simulink model "tasukete"  (R2019b)
settings: Solver=VariableStepAuto  StartTime=0.0  StopTime=60  RelTol=1e-3
values from neighbouring files (symbols this model uses):
  a0 = 1.3    [mf.mat]    (also in model_2r.m; model_Fy.m)
  a1 = -0.0274    [mf.mat]    (also in model_2r.m; model_Fy.m)
  a10 = 0.015    [mf.mat]    (also in model_2r.m; model_Fy.m)
  a11 = 0.00849    [mf.mat]    (also in model_2r.m = 0.0849; model_Fy.m)
  a12 = -0.0103    [mf.mat]    (also in model_2r.m; model_Fy.m)
  a13 = 0.0395    [mf.mat]    (also in model_2r.m; model_Fy.m)
  a2 = 1.05    [mf.mat]    (also in model_2r.m; model_Fy.m)
  a3 = 1.18    [mf.mat]    (also in model_2r.m; model_Fy.m)
  a4 = 7.69    [mf.mat]    (also in model_2r.m; model_Fy.m)
  a5 = 0.009    [mf.mat]    (also in model_2r.m; model_Fy.m)
  a6 = -0.257    [mf.mat]    (also in model_2r.m; model_Fy.m)
  a7 = 0.224    [mf.mat]    (also in model_2r.m; model_Fy.m)
  a8 = 0.025    [mf.mat]    (also in model_2r.m; model_Fy.m)
  a9 = 0.01    [mf.mat]    (also in model_2r.m; model_Fy.m)
  g = 9.81    [mf.mat]    (also in model_2r.m)
  Iz = 1500    [mf.mat]    (also in model_2r.m)
  lf = 1.4    [mf.mat]    (also in model_2r.m = 1.2)
  lr = 1.2    [mf.mat]    (also in model_2r.m = 1.4)
  m = 1200    [mf.mat]    (also in model_2r.m)
  v = 8.33333333333    [mf.mat]    (also in model_2r.m = 100)
libraries: simulink_extras x1, simulink x1
settings Model: Creator=yknc1  LastModifiedBy=Peanatsu
settings SFSimCC: CustomCodeUndefinedFunction=UseInterfaceOnly

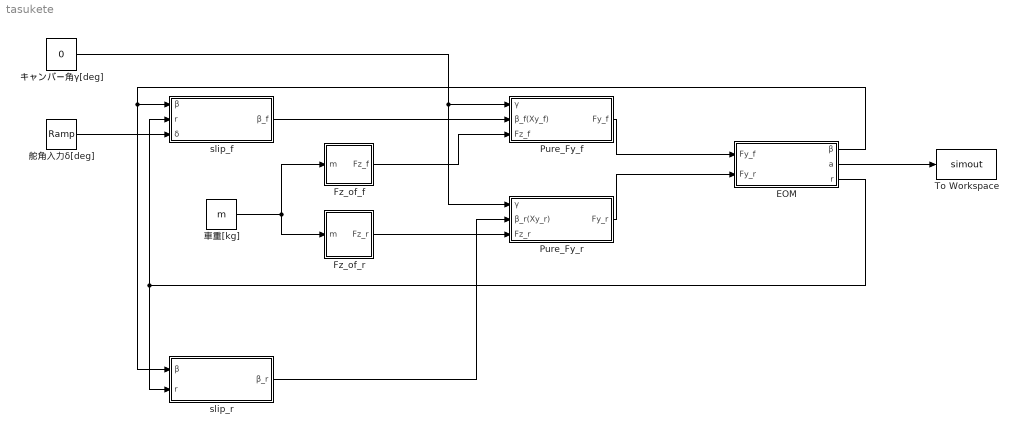
== system tasukete ==
  EOM : Subsystem
  Fz_of_f : Subsystem
  Fz_of_r : Subsystem
  Pure_Fy_f : Subsystem
  Pure_Fy_r : Subsystem
  To Workspace : ToWorkspace  VariableName=simout  SaveFormat=Timeseries  SampleTime=-1
  slip_f : Subsystem
  slip_r : Subsystem
  キャンバー角γ[deg] : Constant  Value=0
  舵角入力δ[deg] : simulink/Sources/Ramp  slope=5  start=0  InitialOutput=1
  車重[kg] : Constant  Value=m
  wires:
  キャンバー角γ[deg]/1 -> Pure_Fy_r/1(γ), Pure_Fy_f/1(γ)
  slip_f/1(β_f) -> Pure_Fy_f/2(β_f(Xy_f))
  slip_r/1(β_r) -> Pure_Fy_r/2(β_r(Xy_r))
  EOM/1(β) -> slip_f/1(β), slip_r/1(β)
  EOM/3(r) -> slip_r/2(r), slip_f/2(r)
  車重[kg]/1 -> Fz_of_r/1(m), Fz_of_f/1(m)
  Fz_of_f/1(Fz_f) -> Pure_Fy_f/3(Fz_f)
  Fz_of_r/1(Fz_r) -> Pure_Fy_r/3(Fz_r)
  Pure_Fy_r/1(Fy_r) -> EOM/2(Fy_r)
  Pure_Fy_f/1(Fy_f) -> EOM/1(Fy_f)
  EOM/2(a) -> To Workspace/1
  舵角入力δ[deg]/1 -> slip_f/3(δ)

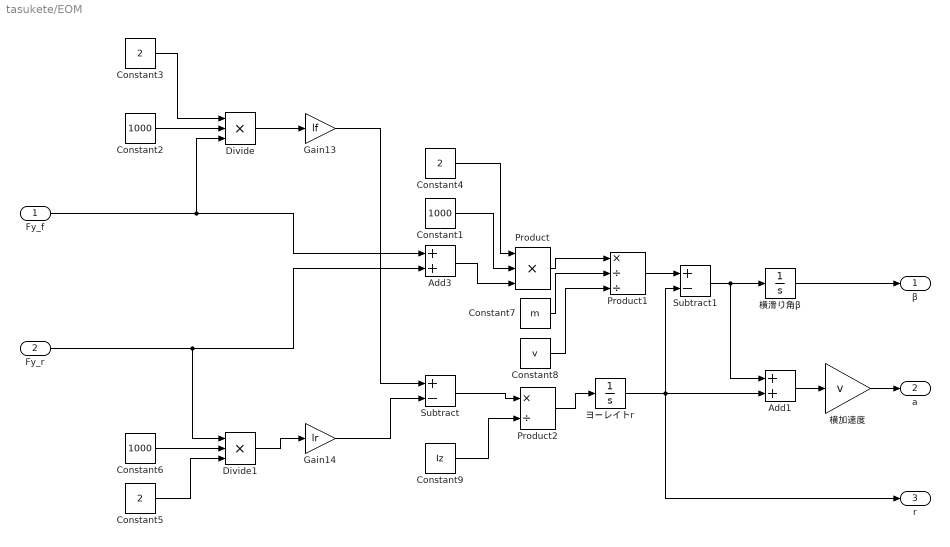
== system tasukete/EOM ==
  Fy_f : Inport
  Fy_r : Inport  Port=2
  Add1 : Sum
  Add3 : Sum
  Constant1 : Constant  Value=1000
  Constant2 : Constant  Value=1000
  Constant3 : Constant  Value=2
  Constant4 : Constant  Value=2
  Constant5 : Constant  Value=2
  Constant6 : Constant  Value=1000
  Constant7 : Constant  Value=m
  Constant8 : Constant  Value=v
  Constant9 : Constant  Value=Iz
  Divide : Product  Inputs=***
  Divide1 : Product  Inputs=***
  Gain13 : Gain  Gain=lf
  Gain14 : Gain  Gain=lr
  Product : Product  Inputs=3
  Product1 : Product  Inputs=*//
  Product2 : Product  Inputs=*/
  Subtract : Sum  Inputs=+-
  Subtract1 : Sum  Inputs=+-
  ヨーレイトr : Integrator
  横加速度 : Gain  Gain=v
  横滑り角β : Integrator
  β : Outport  VectorParamsAs1DForOutWhenUnconnected=off
  a : Outport  Port=2  VectorParamsAs1DForOutWhenUnconnected=off
  r : Outport  Port=3  VectorParamsAs1DForOutWhenUnconnected=off
  wires:
  Subtract1/1 -> Add1/1, 横滑り角β/1
  Constant5/1 -> Divide1/3
  Constant6/1 -> Divide1/2
  ヨーレイトr/1 -> Subtract1/2, Add1/2, r/1
  Divide/1 -> Gain13/1
  Constant1/1 -> Product/2
  Fy_r/1 -> Divide1/1, Add3/2
  Constant4/1 -> Product/1
  Constant2/1 -> Divide/2
  横滑り角β/1 -> β/1
  Add1/1 -> 横加速度/1
  Constant3/1 -> Divide/1
  横加速度/1 -> a/1
  Divide1/1 -> Gain14/1
  Add3/1 -> Product/3
  Gain14/1 -> Subtract/2
  Product1/1 -> Subtract1/1
  Gain13/1 -> Subtract/1
  Fy_f/1 -> Divide/3, Add3/1
  Subtract/1 -> Product2/1
  Product/1 -> Product1/1
  Constant8/1 -> Product1/3
  Constant7/1 -> Product1/2
  Product2/1 -> ヨーレイトr/1
  Constant9/1 -> Product2/2

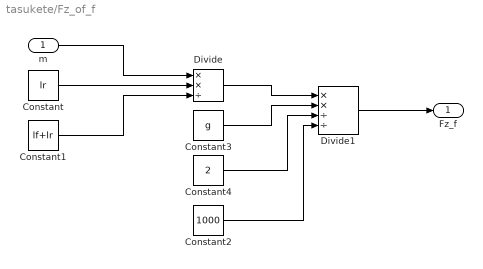
== system tasukete/Fz_of_f ==
  m : Inport
  Constant : Constant  Value=lr
  Constant1 : Constant  Value=lf+lr
  Constant2 : Constant  Value=1000
  Constant3 : Constant  Value=g
  Constant4 : Constant  Value=2
  Divide : Product  Inputs=**/
  Divide1 : Product  Inputs=**//
  Fz_f : Outport  VectorParamsAs1DForOutWhenUnconnected=off
  wires:
  m/1 -> Divide/1
  Constant/1 -> Divide/2
  Constant1/1 -> Divide/3
  Divide/1 -> Divide1/1
  Constant3/1 -> Divide1/2
  Constant4/1 -> Divide1/3
  Constant2/1 -> Divide1/4
  Divide1/1 -> Fz_f/1

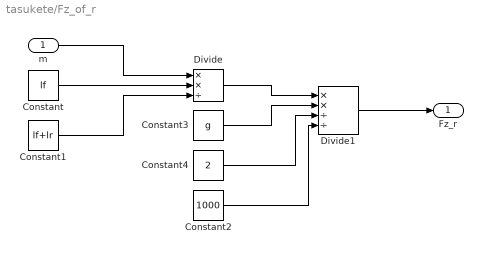
== system tasukete/Fz_of_r ==
  m : Inport
  Constant : Constant  Value=lf
  Constant1 : Constant  Value=lf+lr
  Constant2 : Constant  Value=1000
  Constant3 : Constant  Value=g
  Constant4 : Constant  Value=2
  Divide : Product  Inputs=**/
  Divide1 : Product  Inputs=**//
  Fz_r : Outport  VectorParamsAs1DForOutWhenUnconnected=off
  wires:
  Constant3/1 -> Divide1/2
  Divide1/1 -> Fz_r/1
  Constant/1 -> Divide/2
  Constant2/1 -> Divide1/4
  m/1 -> Divide/1
  Constant4/1 -> Divide1/3
  Constant1/1 -> Divide/3
  Divide/1 -> Divide1/1

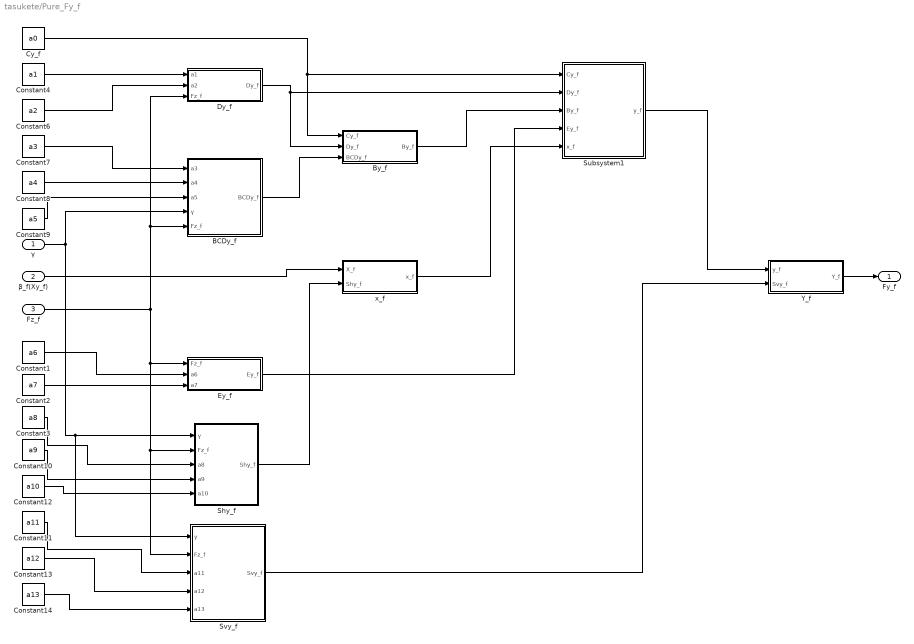
== system tasukete/Pure_Fy_f ==
  γ : Inport
  β_f(Xy_f) : Inport  Port=2
  Fz_f : Inport  Port=3
  BCDy_f : Subsystem
  By_f : Subsystem
  Constant1 : Constant  Value=a6
  Constant10 : Constant  Value=a9
  Constant11 : Constant  Value=a11
  Constant12 : Constant  Value=a10
  Constant13 : Constant  Value=a12
  Constant14 : Constant  Value=a13
  Constant2 : Constant  Value=a7
  Constant3 : Constant  Value=a8
  Constant4 : Constant  Value=a1
  Constant6 : Constant  Value=a2
  Constant7 : Constant  Value=a3
  Constant8 : Constant  Value=a4
  Constant9 : Constant  Value=a5
  Cy_f : Constant  Value=a0
  Dy_f : Subsystem
  Ey_f : Subsystem
  Shy_f : Subsystem
  Subsystem1 : Subsystem
  Svy_f : Subsystem
  Y_f : Subsystem
  x_f : Subsystem
  Fy_f : Outport  VectorParamsAs1DForOutWhenUnconnected=off
  wires:
  Constant4/1 -> Dy_f/1(a1)
  Constant6/1 -> Dy_f/2(a2)
  Fz_f/1 -> BCDy_f/5(Fz_f), Dy_f/3(Fz_f), Ey_f/1(Fz_f), Svy_f/2(Fz_f), Shy_f/2(Fz_f)
  Constant1/1 -> Ey_f/2(a6)
  Constant2/1 -> Ey_f/3(a7)
  γ/1 -> Shy_f/1(γ), Svy_f/1(γ), BCDy_f/4(γ)
  Constant3/1 -> Shy_f/3(a8)
  Constant10/1 -> Shy_f/4(a9)
  Constant12/1 -> Shy_f/5(a10)
  Constant11/1 -> Svy_f/3(a11)
  Constant13/1 -> Svy_f/4(a12)
  Constant14/1 -> Svy_f/5(a13)
  Constant7/1 -> BCDy_f/1(a3)
  Constant8/1 -> BCDy_f/2(a4)
  Constant9/1 -> BCDy_f/3(a5)
  Cy_f/1 -> By_f/1(Cy_f), Subsystem1/1(Cy_f)
  Dy_f/1(Dy_f) -> By_f/2(Dy_f), Subsystem1/2(Dy_f)
  BCDy_f/1(BCDy_f) -> By_f/3(BCDy_f)
  β_f(Xy_f)/1 -> x_f/1(X_f)
  Shy_f/1(Shy_f) -> x_f/2(Shy_f)
  By_f/1(By_f) -> Subsystem1/3(By_f)
  Ey_f/1(Ey_f) -> Subsystem1/4(Ey_f)
  x_f/1(x_f) -> Subsystem1/5(x_f)
  Subsystem1/1(y_f) -> Y_f/1(y_f)
  Svy_f/1(Svy_f) -> Y_f/2(Svy_f)
  Y_f/1(Y_f) -> Fy_f/1

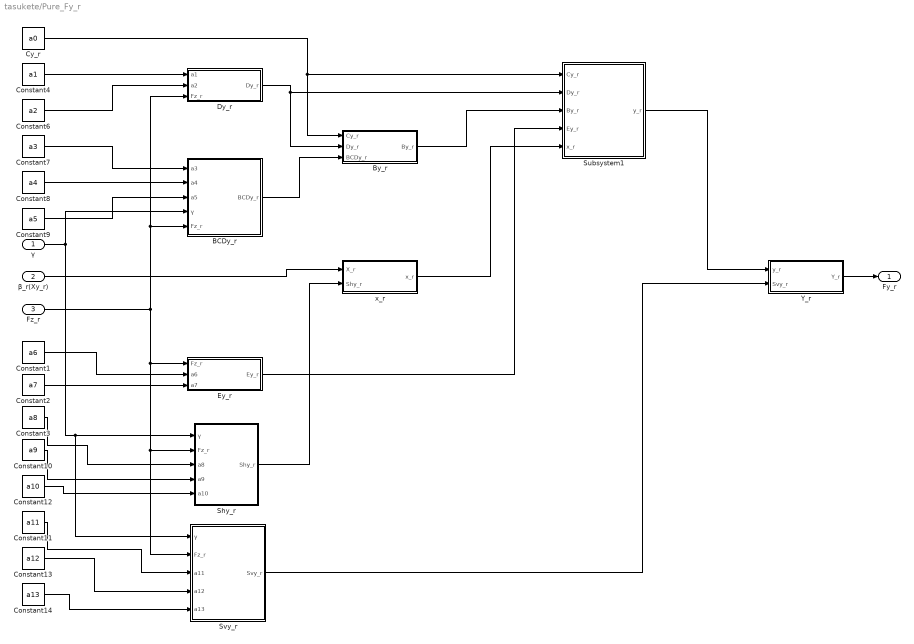
== system tasukete/Pure_Fy_r ==
  γ : Inport
  β_r(Xy_r) : Inport  Port=2
  Fz_r : Inport  Port=3
  BCDy_r : Subsystem
  By_r : Subsystem
  Constant1 : Constant  Value=a6
  Constant10 : Constant  Value=a9
  Constant11 : Constant  Value=a11
  Constant12 : Constant  Value=a10
  Constant13 : Constant  Value=a12
  Constant14 : Constant  Value=a13
  Constant2 : Constant  Value=a7
  Constant3 : Constant  Value=a8
  Constant4 : Constant  Value=a1
  Constant6 : Constant  Value=a2
  Constant7 : Constant  Value=a3
  Constant8 : Constant  Value=a4
  Constant9 : Constant  Value=a5
  Cy_r : Constant  Value=a0
  Dy_r : Subsystem
  Ey_r : Subsystem
  Shy_r : Subsystem
  Subsystem1 : Subsystem
  Svy_r : Subsystem
  Y_r : Subsystem
  x_r : Subsystem
  Fy_r : Outport  VectorParamsAs1DForOutWhenUnconnected=off
  wires:
  Constant4/1 -> Dy_r/1(a1)
  Constant6/1 -> Dy_r/2(a2)
  Fz_r/1 -> BCDy_r/5(Fz_r), Dy_r/3(Fz_r), Ey_r/1(Fz_r), Svy_r/2(Fz_r), Shy_r/2(Fz_r)
  Constant1/1 -> Ey_r/2(a6)
  Constant2/1 -> Ey_r/3(a7)
  γ/1 -> Shy_r/1(γ), Svy_r/1(γ), BCDy_r/4(γ)
  Constant3/1 -> Shy_r/3(a8)
  Constant10/1 -> Shy_r/4(a9)
  Constant12/1 -> Shy_r/5(a10)
  Constant11/1 -> Svy_r/3(a11)
  Constant13/1 -> Svy_r/4(a12)
  Constant14/1 -> Svy_r/5(a13)
  Constant7/1 -> BCDy_r/1(a3)
  Constant8/1 -> BCDy_r/2(a4)
  Constant9/1 -> BCDy_r/3(a5)
  Cy_r/1 -> By_r/1(Cy_r), Subsystem1/1(Cy_r)
  Dy_r/1(Dy_r) -> By_r/2(Dy_r), Subsystem1/2(Dy_r)
  BCDy_r/1(BCDy_r) -> By_r/3(BCDy_r)
  β_r(Xy_r)/1 -> x_r/1(X_r)
  Shy_r/1(Shy_r) -> x_r/2(Shy_r)
  By_r/1(By_r) -> Subsystem1/3(By_r)
  Ey_r/1(Ey_r) -> Subsystem1/4(Ey_r)
  x_r/1(x_r) -> Subsystem1/5(x_r)
  Subsystem1/1(y_r) -> Y_r/1(y_r)
  Svy_r/1(Svy_r) -> Y_r/2(Svy_r)
  Y_r/1(Y_r) -> Fy_r/1

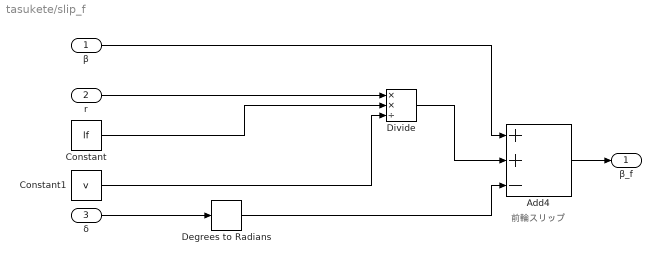
== system tasukete/slip_f ==
  note: 前輪スリップ
  β : Inport
  r : Inport  Port=2
  δ : Inport  Port=3
  Add4 : Sum  Inputs=++-
  Constant : Constant  Value=lf
  Constant1 : Constant  Value=v
  Degrees to Radians : simulink_extras/Transformations/Degrees to Radians
  Divide : Product  Inputs=**/
  β_f : Outport  VectorParamsAs1DForOutWhenUnconnected=off
  wires:
  Add4/1 -> β_f/1
  β/1 -> Add4/1
  δ/1 -> Degrees to Radians/1
  Degrees to Radians/1 -> Add4/3
  r/1 -> Divide/1
  Constant/1 -> Divide/2
  Constant1/1 -> Divide/3
  Divide/1 -> Add4/2

== system tasukete/slip_r ==
  β : Inport
  r : Inport  Port=2
  Constant : Constant  Value=lr
  Constant1 : Constant  Value=v
  Divide : Product  Inputs=**/
  Subtract : Sum  Inputs=+-
  β_r : Outport  VectorParamsAs1DForOutWhenUnconnected=off
  wires:
  β/1 -> Subtract/1
  r/1 -> Divide/1
  Subtract/1 -> β_r/1
  Constant/1 -> Divide/2
  Constant1/1 -> Divide/3
  Divide/1 -> Subtract/2

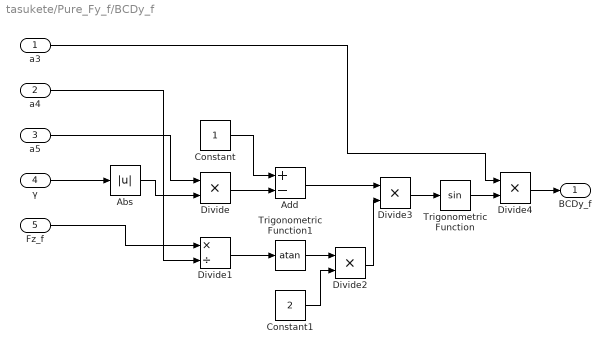
== system tasukete/Pure_Fy_f/BCDy_f ==
  a3 : Inport
  a4 : Inport  Port=2
  a5 : Inport  Port=3
  γ : Inport  Port=4
  Fz_f : Inport  Port=5
  Abs : Abs
  Add : Sum  Inputs=+-
  Constant : Constant
  Constant1 : Constant  Value=2
  Divide{,2..4} (4 alike) : Product  Inputs=**
  Divide1 : Product  Inputs=*/
  Trigonometric Function : Trigonometry
  Trigonometric Function1 : Trigonometry  Operator=atan
  BCDy_f : Outport  VectorParamsAs1DForOutWhenUnconnected=off
  wires:
  γ/1 -> Abs/1
  Abs/1 -> Divide/2
  a5/1 -> Divide/1
  Constant/1 -> Add/1
  Divide/1 -> Add/2
  Fz_f/1 -> Divide1/1
  a4/1 -> Divide1/2
  Divide1/1 -> Trigonometric Function1/1
  Trigonometric Function1/1 -> Divide2/1
  Constant1/1 -> Divide2/2
  Add/1 -> Divide3/1
  Divide2/1 -> Divide3/2
  Divide3/1 -> Trigonometric Function/1
  a3/1 -> Divide4/1
  Trigonometric Function/1 -> Divide4/2
  Divide4/1 -> BCDy_f/1

== system tasukete/Pure_Fy_f/By_f ==
  Cy_f : Inport
  Dy_f : Inport  Port=2
  BCDy_f : Inport  Port=3
  Divide : Product  Inputs=*//
  By_f : Outport  VectorParamsAs1DForOutWhenUnconnected=off
  wires:
  BCDy_f/1 -> Divide/1
  Dy_f/1 -> Divide/2
  Cy_f/1 -> Divide/3
  Divide/1 -> By_f/1

== system tasukete/Pure_Fy_f/Dy_f ==
  a1 : Inport
  a2 : Inport  Port=2
  Fz_f : Inport  Port=3
  Product : Product
  Product1 : Product
  μy_f : Sum
  Dy_f : Outport  VectorParamsAs1DForOutWhenUnconnected=off
  wires:
  a1/1 -> Product/1
  Fz_f/1 -> Product1/2, Product/2
  a2/1 -> μy_f/1
  Product/1 -> μy_f/2
  μy_f/1 -> Product1/1
  Product1/1 -> Dy_f/1

== system tasukete/Pure_Fy_f/Ey_f ==
  Fz_f : Inport
  a6 : Inport  Port=2
  a7 : Inport  Port=3
  Add : Sum
  Product : Product
  Ey_f : Outport  VectorParamsAs1DForOutWhenUnconnected=off
  wires:
  Fz_f/1 -> Product/1
  a6/1 -> Product/2
  Product/1 -> Add/1
  a7/1 -> Add/2
  Add/1 -> Ey_f/1

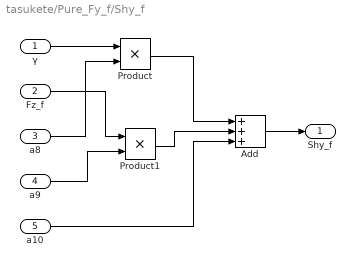
== system tasukete/Pure_Fy_f/Shy_f ==
  γ : Inport
  Fz_f : Inport  Port=2
  a8 : Inport  Port=3
  a9 : Inport  Port=4
  a10 : Inport  Port=5
  Add : Sum  Inputs=+++
  Product : Product
  Product1 : Product
  Shy_f : Outport  VectorParamsAs1DForOutWhenUnconnected=off
  wires:
  γ/1 -> Product/1
  a8/1 -> Product/2
  a9/1 -> Product1/2
  Fz_f/1 -> Product1/1
  a10/1 -> Add/3
  Product1/1 -> Add/2
  Product/1 -> Add/1
  Add/1 -> Shy_f/1

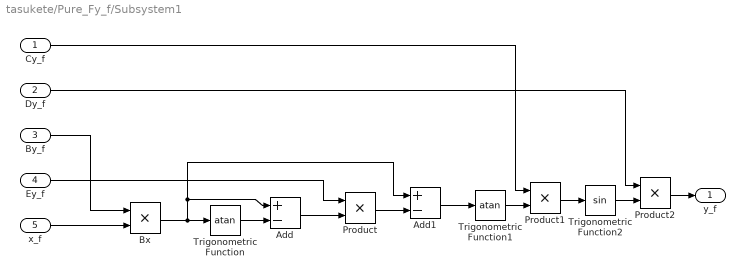
== system tasukete/Pure_Fy_f/Subsystem1 ==
  Cy_f : Inport
  Dy_f : Inport  Port=2
  By_f : Inport  Port=3
  Ey_f : Inport  Port=4
  x_f : Inport  Port=5
  Add : Sum  Inputs=+-
  Add1 : Sum  Inputs=+-
  Bx : Product
  Product : Product
  Product1 : Product
  Product2 : Product
  Trigonometric Function : Trigonometry  Operator=atan
  Trigonometric Function1 : Trigonometry  Operator=atan
  Trigonometric Function2 : Trigonometry
  y_f : Outport  VectorParamsAs1DForOutWhenUnconnected=off
  wires:
  x_f/1 -> Bx/2
  By_f/1 -> Bx/1
  Bx/1 -> Add1/1, Add/1, Trigonometric Function/1
  Trigonometric Function/1 -> Add/2
  Add/1 -> Product/2
  Ey_f/1 -> Product/1
  Product/1 -> Add1/2
  Add1/1 -> Trigonometric Function1/1
  Trigonometric Function1/1 -> Product1/2
  Cy_f/1 -> Product1/1
  Product1/1 -> Trigonometric Function2/1
  Trigonometric Function2/1 -> Product2/2
  Dy_f/1 -> Product2/1
  Product2/1 -> y_f/1

== system tasukete/Pure_Fy_f/Svy_f ==
  γ : Inport
  Fz_f : Inport  Port=2
  a11 : Inport  Port=3
  a12 : Inport  Port=4
  a13 : Inport  Port=5
  Add : Sum  Inputs=+++
  Product : Product  Inputs=3
  Product1 : Product
  Svy_f : Outport  VectorParamsAs1DForOutWhenUnconnected=off
  wires:
  γ/1 -> Product/1
  Fz_f/1 -> Product1/1, Product/2
  a11/1 -> Product/3
  a12/1 -> Product1/2
  Product/1 -> Add/1
  Product1/1 -> Add/2
  a13/1 -> Add/3
  Add/1 -> Svy_f/1

== system tasukete/Pure_Fy_f/Y_f ==
  y_f : Inport
  Svy_f : Inport  Port=2
  Add : Sum
  Y_f : Outport  VectorParamsAs1DForOutWhenUnconnected=off
  wires:
  Add/1 -> Y_f/1
  Svy_f/1 -> Add/2
  y_f/1 -> Add/1

== system tasukete/Pure_Fy_f/x_f ==
  X_f : Inport
  Shy_f : Inport  Port=2
  Add : Sum
  x_f : Outport  VectorParamsAs1DForOutWhenUnconnected=off
  wires:
  X_f/1 -> Add/1
  Shy_f/1 -> Add/2
  Add/1 -> x_f/1

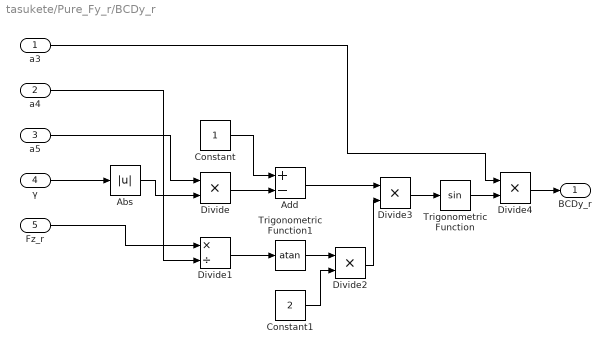
== system tasukete/Pure_Fy_r/BCDy_r ==
  a3 : Inport
  a4 : Inport  Port=2
  a5 : Inport  Port=3
  γ : Inport  Port=4
  Fz_r : Inport  Port=5
  Abs : Abs
  Add : Sum  Inputs=+-
  Constant : Constant
  Constant1 : Constant  Value=2
  Divide{,2..4} (4 alike) : Product  Inputs=**
  Divide1 : Product  Inputs=*/
  Trigonometric Function : Trigonometry
  Trigonometric Function1 : Trigonometry  Operator=atan
  BCDy_r : Outport  VectorParamsAs1DForOutWhenUnconnected=off
  wires:
  γ/1 -> Abs/1
  Abs/1 -> Divide/2
  a5/1 -> Divide/1
  Constant/1 -> Add/1
  Divide/1 -> Add/2
  Fz_r/1 -> Divide1/1
  a4/1 -> Divide1/2
  Divide1/1 -> Trigonometric Function1/1
  Trigonometric Function1/1 -> Divide2/1
  Constant1/1 -> Divide2/2
  Add/1 -> Divide3/1
  Divide2/1 -> Divide3/2
  Divide3/1 -> Trigonometric Function/1
  a3/1 -> Divide4/1
  Trigonometric Function/1 -> Divide4/2
  Divide4/1 -> BCDy_r/1

== system tasukete/Pure_Fy_r/By_r ==
  Cy_r : Inport
  Dy_r : Inport  Port=2
  BCDy_r : Inport  Port=3
  Divide : Product  Inputs=*//
  By_r : Outport  VectorParamsAs1DForOutWhenUnconnected=off
  wires:
  BCDy_r/1 -> Divide/1
  Dy_r/1 -> Divide/2
  Cy_r/1 -> Divide/3
  Divide/1 -> By_r/1

== system tasukete/Pure_Fy_r/Dy_r ==
  a1 : Inport
  a2 : Inport  Port=2
  Fz_r : Inport  Port=3
  Product : Product
  Product1 : Product
  μy_r : Sum
  Dy_r : Outport  VectorParamsAs1DForOutWhenUnconnected=off
  wires:
  a1/1 -> Product/1
  Fz_r/1 -> Product1/2, Product/2
  a2/1 -> μy_r/1
  Product/1 -> μy_r/2
  μy_r/1 -> Product1/1
  Product1/1 -> Dy_r/1

== system tasukete/Pure_Fy_r/Ey_r ==
  Fz_r : Inport
  a6 : Inport  Port=2
  a7 : Inport  Port=3
  Add : Sum
  Product : Product
  Ey_r : Outport  VectorParamsAs1DForOutWhenUnconnected=off
  wires:
  Fz_r/1 -> Product/1
  a6/1 -> Product/2
  Product/1 -> Add/1
  a7/1 -> Add/2
  Add/1 -> Ey_r/1

== system tasukete/Pure_Fy_r/Shy_r ==
  γ : Inport
  Fz_r : Inport  Port=2
  a8 : Inport  Port=3
  a9 : Inport  Port=4
  a10 : Inport  Port=5
  Add : Sum  Inputs=+++
  Product : Product
  Product1 : Product
  Shy_r : Outport  VectorParamsAs1DForOutWhenUnconnected=off
  wires:
  γ/1 -> Product/1
  a8/1 -> Product/2
  a9/1 -> Product1/2
  Fz_r/1 -> Product1/1
  a10/1 -> Add/3
  Product1/1 -> Add/2
  Product/1 -> Add/1
  Add/1 -> Shy_r/1

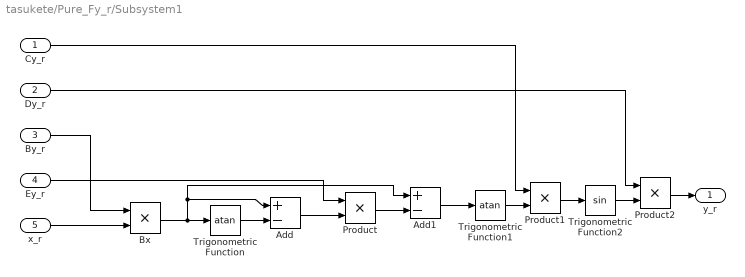
== system tasukete/Pure_Fy_r/Subsystem1 ==
  Cy_r : Inport
  Dy_r : Inport  Port=2
  By_r : Inport  Port=3
  Ey_r : Inport  Port=4
  x_r : Inport  Port=5
  Add : Sum  Inputs=+-
  Add1 : Sum  Inputs=+-
  Bx : Product
  Product : Product
  Product1 : Product
  Product2 : Product
  Trigonometric Function : Trigonometry  Operator=atan
  Trigonometric Function1 : Trigonometry  Operator=atan
  Trigonometric Function2 : Trigonometry
  y_r : Outport  VectorParamsAs1DForOutWhenUnconnected=off
  wires:
  x_r/1 -> Bx/2
  By_r/1 -> Bx/1
  Bx/1 -> Add1/1, Add/1, Trigonometric Function/1
  Trigonometric Function/1 -> Add/2
  Add/1 -> Product/2
  Ey_r/1 -> Product/1
  Product/1 -> Add1/2
  Add1/1 -> Trigonometric Function1/1
  Trigonometric Function1/1 -> Product1/2
  Cy_r/1 -> Product1/1
  Product1/1 -> Trigonometric Function2/1
  Trigonometric Function2/1 -> Product2/2
  Dy_r/1 -> Product2/1
  Product2/1 -> y_r/1

== system tasukete/Pure_Fy_r/Svy_r ==
  γ : Inport
  Fz_r : Inport  Port=2
  a11 : Inport  Port=3
  a12 : Inport  Port=4
  a13 : Inport  Port=5
  Add : Sum  Inputs=+++
  Product : Product  Inputs=3
  Product1 : Product
  Svy_r : Outport  VectorParamsAs1DForOutWhenUnconnected=off
  wires:
  γ/1 -> Product/1
  Fz_r/1 -> Product1/1, Product/2
  a11/1 -> Product/3
  a12/1 -> Product1/2
  Product/1 -> Add/1
  Product1/1 -> Add/2
  a13/1 -> Add/3
  Add/1 -> Svy_r/1

== system tasukete/Pure_Fy_r/Y_r ==
  y_r : Inport
  Svy_r : Inport  Port=2
  Add : Sum
  Y_r : Outport  VectorParamsAs1DForOutWhenUnconnected=off
  wires:
  Add/1 -> Y_r/1
  Svy_r/1 -> Add/2
  y_r/1 -> Add/1

== system tasukete/Pure_Fy_r/x_r ==
  X_r : Inport
  Shy_r : Inport  Port=2
  Add : Sum
  x_r : Outport  VectorParamsAs1DForOutWhenUnconnected=off
  wires:
  X_r/1 -> Add/1
  Shy_r/1 -> Add/2
  Add/1 -> x_r/1
